simulink model "Modelling_Induction"  (R2016a)
settings: Solver=VariableStepAuto  StartTime=0.0  StopTime=10.0  RelTol=1e-3
settings Model: Creator=Mohamed elghazali  LastModifiedBy=Mohamed elghazali

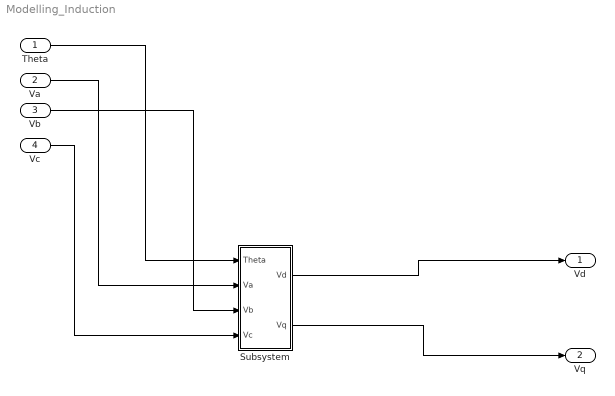
== system Modelling_Induction ==
  Theta : Inport
  Va : Inport  Port=2
  Vb : Inport  Port=3
  Vc : Inport  Port=4
  Subsystem : Subsystem
  Vd : Outport
  Vq : Outport  Port=2
  wires:
  Theta/1 -> Subsystem/1(Theta)
  Va/1 -> Subsystem/2(Va)
  Vb/1 -> Subsystem/3(Vb)
  Vc/1 -> Subsystem/4(Vc)
  Subsystem/1(Vd) -> Vd/1
  Subsystem/2(Vq) -> Vq/1

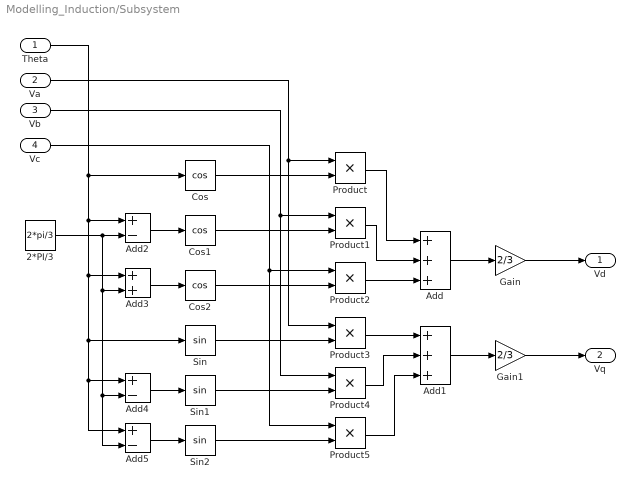
== system Modelling_Induction/Subsystem ==
  Theta : Inport
  Va : Inport  Port=2
  Vb : Inport  Port=3
  Vc : Inport  Port=4
  2*PI/3 : Constant  Value=2*pi/3
  Add : Sum  Inputs=+++
  Add1 : Sum  Inputs=+++
  Add2 : Sum  Inputs=+-
  Add3 : Sum
  Add4 : Sum  Inputs=+-
  Add5 : Sum  Inputs=+-
  Cos : Trigonometry  Operator=cos
  Cos1 : Trigonometry  Operator=cos
  Cos2 : Trigonometry  Operator=cos
  Gain : Gain  Gain=2/3
  Gain1 : Gain  Gain=2/3
  Product{,1..5} (6 alike) : Product
  Sin : Trigonometry
  Sin1 : Trigonometry
  Sin2 : Trigonometry
  Vd : Outport
  Vq : Outport  Port=2
  wires:
  Product5/1 -> Add1/3
  Product3/1 -> Add1/1
  Product4/1 -> Add1/2
  Product2/1 -> Add/3
  Gain1/1 -> Vq/1
  Add/1 -> Gain/1
  Add1/1 -> Gain1/1
  Product1/1 -> Add/2
  Product/1 -> Add/1
  Gain/1 -> Vd/1
  Vb/1 -> Product4/1, Product1/1
  Sin1/1 -> Product4/2
  Add4/1 -> Sin1/1
  Sin/1 -> Product3/2
  Cos2/1 -> Product2/2
  Add3/1 -> Cos2/1
  Theta/1 -> Cos/1, Add3/1, Sin/1, Add4/1, Add5/1, Add2/1
  Cos/1 -> Product/2
  Cos1/1 -> Product1/2
  Add2/1 -> Cos1/1
  Add5/1 -> Sin2/1
  2*PI/3/1 -> Add3/2, Add5/2, Add4/2, Add2/2
  Va/1 -> Product3/1, Product/1
  Vc/1 -> Product5/1, Product2/1
  Sin2/1 -> Product5/2
